simulink model "unrolled_pipelined_parallel"  (R2015b)
settings: Solver=FixedStepDiscrete  SolverMode=SingleTasking  StartTime=0.0  StopTime=10.0  RelTol=1e-3
undefined symbols (not defined in the file or in its folder): a, b
libraries: shlslibv1 x8781
(part 14 of 32)

== system unrolled_pipelined_parallel/Subsystem/Subsystem3/SB_rs_MIX_COLUMN/Subsystem2/multby2 ==
  In1 : Inport
  Binary Logic : shlslibv1/Math Functions/Binary Logic  syn_binlog_exp=a^b  synBlockType=primitive  synLatency=0  synBlockId=13
  Comparator : shlslibv1/Math Functions/Comparator  syn_comp_opr=a==b  syn_comp_const=off  syn_comp_val=0  syn_en_se=off  synBlockType=primitive  synLatency=0  synBlockId=14
  Constant : shlslibv1/Sources/Constant  syn_cst_val=1  syn_cst_format=Automatic  syn_cst_wl=1  syn_cst_fl=0  syn_cst_dt=unsigned  syn_cst_rnd=on  syn_cst_st=-1  synBlockType=primitive  synLatency=0  synBlockId=15
  Constant1 : shlslibv1/Sources/Constant  syn_cst_val=1  syn_cst_format=Automatic  syn_cst_wl=1  syn_cst_fl=0  syn_cst_dt=unsigned  syn_cst_rnd=on  syn_cst_st=-1  synBlockType=primitive  synLatency=0  synBlockId=15
  Constant2 : shlslibv1/Sources/Constant  syn_cst_val=27  syn_cst_format=Specify  syn_cst_wl=8  syn_cst_fl=0  syn_cst_dt=unsigned  syn_cst_rnd=on  syn_cst_st=-1  synBlockType=primitive  synLatency=0  synBlockId=15
  Extract : shlslibv1/Signal Operations/Extract  syn_extract_vec=[7]  synBlockType=primitive  synLatency=0  synBlockId=17
  Mux : shlslibv1/Signal Operations/Mux  syn_in_nb=2  syn_out_f=Full Precision  syn_out_wl=16  syn_out_fl=8  syn_out_dt=signed  syn_en_se=off  synBlockType=primitive  synLatency=0  synBlockId=16
  Shifter : shlslibv1/Math Functions/Shifter  syn_shifter_opr=<<  syn_out_f=Automatic  syn_out_wl=16  syn_out_fl=8  syn_out_dt=signed  synBlockType=primitive  synLatency=0  synBlockId=12
  Out1 : Outport
  wires:
  Extract/1 -> Comparator/1
  In1/1 -> Shifter/1, Extract/1
  Constant/1 -> Shifter/2
  Constant1/1 -> Comparator/2
  Shifter/1 -> Mux/2, Binary Logic/1
  Comparator/1 -> Mux/1
  Mux/1 -> Out1/1
  Binary Logic/1 -> Mux/3
  Constant2/1 -> Binary Logic/2

== system unrolled_pipelined_parallel/Subsystem/Subsystem3/SB_rs_MIX_COLUMN/Subsystem2/multby3 ==
  In1 : Inport
  Binary Logic : shlslibv1/Math Functions/Binary Logic  syn_binlog_exp=a^b  synBlockType=primitive  synLatency=0  synBlockId=13
  Comparator : shlslibv1/Math Functions/Comparator  syn_comp_opr=a==b  syn_comp_const=off  syn_comp_val=0  syn_en_se=off  synBlockType=primitive  synLatency=0  synBlockId=14
  Constant : shlslibv1/Sources/Constant  syn_cst_val=1  syn_cst_format=Automatic  syn_cst_wl=1  syn_cst_fl=0  syn_cst_dt=unsigned  syn_cst_rnd=on  syn_cst_st=-1  synBlockType=primitive  synLatency=0  synBlockId=15
  Constant1 : shlslibv1/Sources/Constant  syn_cst_val=1  syn_cst_format=Automatic  syn_cst_wl=1  syn_cst_fl=0  syn_cst_dt=unsigned  syn_cst_rnd=on  syn_cst_st=-1  synBlockType=primitive  synLatency=0  synBlockId=15
  Constant2 : shlslibv1/Sources/Constant  syn_cst_val=27  syn_cst_format=Specify  syn_cst_wl=8  syn_cst_fl=0  syn_cst_dt=unsigned  syn_cst_rnd=on  syn_cst_st=-1  synBlockType=primitive  synLatency=0  synBlockId=15
  Extract : shlslibv1/Signal Operations/Extract  syn_extract_vec=[7]  synBlockType=primitive  synLatency=0  synBlockId=17
  Mux : shlslibv1/Signal Operations/Mux  syn_in_nb=2  syn_out_f=Full Precision  syn_out_wl=16  syn_out_fl=8  syn_out_dt=signed  syn_en_se=off  synBlockType=primitive  synLatency=0  synBlockId=16
  Shifter : shlslibv1/Math Functions/Shifter  syn_shifter_opr=<<  syn_out_f=Automatic  syn_out_wl=16  syn_out_fl=8  syn_out_dt=signed  synBlockType=primitive  synLatency=0  synBlockId=12
  Out1 : Outport
  wires:
  Extract/1 -> Comparator/1
  In1/1 -> Shifter/1, Extract/1
  Constant/1 -> Shifter/2
  Constant1/1 -> Comparator/2
  Shifter/1 -> Mux/2, Binary Logic/1
  Comparator/1 -> Mux/1
  Mux/1 -> Out1/1
  Binary Logic/1 -> Mux/3
  Constant2/1 -> Binary Logic/2

== system unrolled_pipelined_parallel/Subsystem/Subsystem3/SB_rs_MIX_COLUMN/Subsystem2/multby4 ==
  In1 : Inport
  Binary Logic : shlslibv1/Math Functions/Binary Logic  syn_binlog_exp=a^b  synBlockType=primitive  synLatency=0  synBlockId=13
  Comparator : shlslibv1/Math Functions/Comparator  syn_comp_opr=a==b  syn_comp_const=off  syn_comp_val=0  syn_en_se=off  synBlockType=primitive  synLatency=0  synBlockId=14
  Constant : shlslibv1/Sources/Constant  syn_cst_val=1  syn_cst_format=Automatic  syn_cst_wl=1  syn_cst_fl=0  syn_cst_dt=unsigned  syn_cst_rnd=on  syn_cst_st=-1  synBlockType=primitive  synLatency=0  synBlockId=15
  Constant1 : shlslibv1/Sources/Constant  syn_cst_val=1  syn_cst_format=Automatic  syn_cst_wl=1  syn_cst_fl=0  syn_cst_dt=unsigned  syn_cst_rnd=on  syn_cst_st=-1  synBlockType=primitive  synLatency=0  synBlockId=15
  Constant2 : shlslibv1/Sources/Constant  syn_cst_val=27  syn_cst_format=Specify  syn_cst_wl=8  syn_cst_fl=0  syn_cst_dt=unsigned  syn_cst_rnd=on  syn_cst_st=-1  synBlockType=primitive  synLatency=0  synBlockId=15
  Extract : shlslibv1/Signal Operations/Extract  syn_extract_vec=[7]  synBlockType=primitive  synLatency=0  synBlockId=17
  Mux : shlslibv1/Signal Operations/Mux  syn_in_nb=2  syn_out_f=Full Precision  syn_out_wl=16  syn_out_fl=8  syn_out_dt=signed  syn_en_se=off  synBlockType=primitive  synLatency=0  synBlockId=16
  Shifter : shlslibv1/Math Functions/Shifter  syn_shifter_opr=<<  syn_out_f=Automatic  syn_out_wl=16  syn_out_fl=8  syn_out_dt=signed  synBlockType=primitive  synLatency=0  synBlockId=12
  Out1 : Outport
  wires:
  Extract/1 -> Comparator/1
  In1/1 -> Shifter/1, Extract/1
  Constant/1 -> Shifter/2
  Constant1/1 -> Comparator/2
  Shifter/1 -> Mux/2, Binary Logic/1
  Comparator/1 -> Mux/1
  Mux/1 -> Out1/1
  Binary Logic/1 -> Mux/3
  Constant2/1 -> Binary Logic/2

== system unrolled_pipelined_parallel/Subsystem/Subsystem3/SB_rs_MIX_COLUMN/Subsystem2/multby5 ==
  In1 : Inport
  Binary Logic : shlslibv1/Math Functions/Binary Logic  syn_binlog_exp=a^b  synBlockType=primitive  synLatency=0  synBlockId=13
  Comparator : shlslibv1/Math Functions/Comparator  syn_comp_opr=a==b  syn_comp_const=off  syn_comp_val=0  syn_en_se=off  synBlockType=primitive  synLatency=0  synBlockId=14
  Constant : shlslibv1/Sources/Constant  syn_cst_val=1  syn_cst_format=Automatic  syn_cst_wl=1  syn_cst_fl=0  syn_cst_dt=unsigned  syn_cst_rnd=on  syn_cst_st=-1  synBlockType=primitive  synLatency=0  synBlockId=15
  Constant1 : shlslibv1/Sources/Constant  syn_cst_val=1  syn_cst_format=Automatic  syn_cst_wl=1  syn_cst_fl=0  syn_cst_dt=unsigned  syn_cst_rnd=on  syn_cst_st=-1  synBlockType=primitive  synLatency=0  synBlockId=15
  Constant2 : shlslibv1/Sources/Constant  syn_cst_val=27  syn_cst_format=Specify  syn_cst_wl=8  syn_cst_fl=0  syn_cst_dt=unsigned  syn_cst_rnd=on  syn_cst_st=-1  synBlockType=primitive  synLatency=0  synBlockId=15
  Extract : shlslibv1/Signal Operations/Extract  syn_extract_vec=[7]  synBlockType=primitive  synLatency=0  synBlockId=17
  Mux : shlslibv1/Signal Operations/Mux  syn_in_nb=2  syn_out_f=Full Precision  syn_out_wl=16  syn_out_fl=8  syn_out_dt=signed  syn_en_se=off  synBlockType=primitive  synLatency=0  synBlockId=16
  Shifter : shlslibv1/Math Functions/Shifter  syn_shifter_opr=<<  syn_out_f=Automatic  syn_out_wl=16  syn_out_fl=8  syn_out_dt=signed  synBlockType=primitive  synLatency=0  synBlockId=12
  Out1 : Outport
  wires:
  Extract/1 -> Comparator/1
  In1/1 -> Shifter/1, Extract/1
  Constant/1 -> Shifter/2
  Constant1/1 -> Comparator/2
  Shifter/1 -> Mux/2, Binary Logic/1
  Comparator/1 -> Mux/1
  Mux/1 -> Out1/1
  Binary Logic/1 -> Mux/3
  Constant2/1 -> Binary Logic/2

== system unrolled_pipelined_parallel/Subsystem/Subsystem3/SB_rs_MIX_COLUMN/Subsystem2/multby6 ==
  In1 : Inport
  Binary Logic : shlslibv1/Math Functions/Binary Logic  syn_binlog_exp=a^b  synBlockType=primitive  synLatency=0  synBlockId=13
  Comparator : shlslibv1/Math Functions/Comparator  syn_comp_opr=a==b  syn_comp_const=off  syn_comp_val=0  syn_en_se=off  synBlockType=primitive  synLatency=0  synBlockId=14
  Constant : shlslibv1/Sources/Constant  syn_cst_val=1  syn_cst_format=Automatic  syn_cst_wl=1  syn_cst_fl=0  syn_cst_dt=unsigned  syn_cst_rnd=on  syn_cst_st=-1  synBlockType=primitive  synLatency=0  synBlockId=15
  Constant1 : shlslibv1/Sources/Constant  syn_cst_val=1  syn_cst_format=Automatic  syn_cst_wl=1  syn_cst_fl=0  syn_cst_dt=unsigned  syn_cst_rnd=on  syn_cst_st=-1  synBlockType=primitive  synLatency=0  synBlockId=15
  Constant2 : shlslibv1/Sources/Constant  syn_cst_val=27  syn_cst_format=Specify  syn_cst_wl=8  syn_cst_fl=0  syn_cst_dt=unsigned  syn_cst_rnd=on  syn_cst_st=-1  synBlockType=primitive  synLatency=0  synBlockId=15
  Extract : shlslibv1/Signal Operations/Extract  syn_extract_vec=[7]  synBlockType=primitive  synLatency=0  synBlockId=17
  Mux : shlslibv1/Signal Operations/Mux  syn_in_nb=2  syn_out_f=Full Precision  syn_out_wl=16  syn_out_fl=8  syn_out_dt=signed  syn_en_se=off  synBlockType=primitive  synLatency=0  synBlockId=16
  Shifter : shlslibv1/Math Functions/Shifter  syn_shifter_opr=<<  syn_out_f=Automatic  syn_out_wl=16  syn_out_fl=8  syn_out_dt=signed  synBlockType=primitive  synLatency=0  synBlockId=12
  Out1 : Outport
  wires:
  Extract/1 -> Comparator/1
  In1/1 -> Shifter/1, Extract/1
  Constant/1 -> Shifter/2
  Constant1/1 -> Comparator/2
  Shifter/1 -> Mux/2, Binary Logic/1
  Comparator/1 -> Mux/1
  Mux/1 -> Out1/1
  Binary Logic/1 -> Mux/3
  Constant2/1 -> Binary Logic/2

== system unrolled_pipelined_parallel/Subsystem/Subsystem3/SB_rs_MIX_COLUMN/Subsystem2/multby7 ==
  In1 : Inport
  Binary Logic : shlslibv1/Math Functions/Binary Logic  syn_binlog_exp=a^b  synBlockType=primitive  synLatency=0  synBlockId=13
  Comparator : shlslibv1/Math Functions/Comparator  syn_comp_opr=a==b  syn_comp_const=off  syn_comp_val=0  syn_en_se=off  synBlockType=primitive  synLatency=0  synBlockId=14
  Constant : shlslibv1/Sources/Constant  syn_cst_val=1  syn_cst_format=Automatic  syn_cst_wl=1  syn_cst_fl=0  syn_cst_dt=unsigned  syn_cst_rnd=on  syn_cst_st=-1  synBlockType=primitive  synLatency=0  synBlockId=15
  Constant1 : shlslibv1/Sources/Constant  syn_cst_val=1  syn_cst_format=Automatic  syn_cst_wl=1  syn_cst_fl=0  syn_cst_dt=unsigned  syn_cst_rnd=on  syn_cst_st=-1  synBlockType=primitive  synLatency=0  synBlockId=15
  Constant2 : shlslibv1/Sources/Constant  syn_cst_val=27  syn_cst_format=Specify  syn_cst_wl=8  syn_cst_fl=0  syn_cst_dt=unsigned  syn_cst_rnd=on  syn_cst_st=-1  synBlockType=primitive  synLatency=0  synBlockId=15
  Extract : shlslibv1/Signal Operations/Extract  syn_extract_vec=[7]  synBlockType=primitive  synLatency=0  synBlockId=17
  Mux : shlslibv1/Signal Operations/Mux  syn_in_nb=2  syn_out_f=Full Precision  syn_out_wl=16  syn_out_fl=8  syn_out_dt=signed  syn_en_se=off  synBlockType=primitive  synLatency=0  synBlockId=16
  Shifter : shlslibv1/Math Functions/Shifter  syn_shifter_opr=<<  syn_out_f=Automatic  syn_out_wl=16  syn_out_fl=8  syn_out_dt=signed  synBlockType=primitive  synLatency=0  synBlockId=12
  Out1 : Outport
  wires:
  Extract/1 -> Comparator/1
  In1/1 -> Shifter/1, Extract/1
  Constant/1 -> Shifter/2
  Constant1/1 -> Comparator/2
  Shifter/1 -> Mux/2, Binary Logic/1
  Comparator/1 -> Mux/1
  Mux/1 -> Out1/1
  Binary Logic/1 -> Mux/3
  Constant2/1 -> Binary Logic/2

== system unrolled_pipelined_parallel/Subsystem/Subsystem3/SB_rs_MIX_COLUMN/Subsystem2/multby8 ==
  In1 : Inport
  Binary Logic : shlslibv1/Math Functions/Binary Logic  syn_binlog_exp=a^b  synBlockType=primitive  synLatency=0  synBlockId=13
  Comparator : shlslibv1/Math Functions/Comparator  syn_comp_opr=a==b  syn_comp_const=off  syn_comp_val=0  syn_en_se=off  synBlockType=primitive  synLatency=0  synBlockId=14
  Constant : shlslibv1/Sources/Constant  syn_cst_val=1  syn_cst_format=Automatic  syn_cst_wl=1  syn_cst_fl=0  syn_cst_dt=unsigned  syn_cst_rnd=on  syn_cst_st=-1  synBlockType=primitive  synLatency=0  synBlockId=15
  Constant1 : shlslibv1/Sources/Constant  syn_cst_val=1  syn_cst_format=Automatic  syn_cst_wl=1  syn_cst_fl=0  syn_cst_dt=unsigned  syn_cst_rnd=on  syn_cst_st=-1  synBlockType=primitive  synLatency=0  synBlockId=15
  Constant2 : shlslibv1/Sources/Constant  syn_cst_val=27  syn_cst_format=Specify  syn_cst_wl=8  syn_cst_fl=0  syn_cst_dt=unsigned  syn_cst_rnd=on  syn_cst_st=-1  synBlockType=primitive  synLatency=0  synBlockId=15
  Extract : shlslibv1/Signal Operations/Extract  syn_extract_vec=[7]  synBlockType=primitive  synLatency=0  synBlockId=17
  Mux : shlslibv1/Signal Operations/Mux  syn_in_nb=2  syn_out_f=Full Precision  syn_out_wl=16  syn_out_fl=8  syn_out_dt=signed  syn_en_se=off  synBlockType=primitive  synLatency=0  synBlockId=16
  Shifter : shlslibv1/Math Functions/Shifter  syn_shifter_opr=<<  syn_out_f=Automatic  syn_out_wl=16  syn_out_fl=8  syn_out_dt=signed  synBlockType=primitive  synLatency=0  synBlockId=12
  Out1 : Outport
  wires:
  Extract/1 -> Comparator/1
  In1/1 -> Shifter/1, Extract/1
  Constant/1 -> Shifter/2
  Constant1/1 -> Comparator/2
  Shifter/1 -> Mux/2, Binary Logic/1
  Comparator/1 -> Mux/1
  Mux/1 -> Out1/1
  Binary Logic/1 -> Mux/3
  Constant2/1 -> Binary Logic/2

== system unrolled_pipelined_parallel/Subsystem/Subsystem3/SB_rs_MIX_COLUMN/Subsystem3/multby1 ==
  In1 : Inport
  Binary Logic : shlslibv1/Math Functions/Binary Logic  syn_binlog_exp=a^b  synBlockType=primitive  synLatency=0  synBlockId=13
  Comparator : shlslibv1/Math Functions/Comparator  syn_comp_opr=a==b  syn_comp_const=off  syn_comp_val=0  syn_en_se=off  synBlockType=primitive  synLatency=0  synBlockId=14
  Constant : shlslibv1/Sources/Constant  syn_cst_val=1  syn_cst_format=Automatic  syn_cst_wl=1  syn_cst_fl=0  syn_cst_dt=unsigned  syn_cst_rnd=on  syn_cst_st=-1  synBlockType=primitive  synLatency=0  synBlockId=15
  Constant1 : shlslibv1/Sources/Constant  syn_cst_val=1  syn_cst_format=Automatic  syn_cst_wl=1  syn_cst_fl=0  syn_cst_dt=unsigned  syn_cst_rnd=on  syn_cst_st=-1  synBlockType=primitive  synLatency=0  synBlockId=15
  Constant2 : shlslibv1/Sources/Constant  syn_cst_val=27  syn_cst_format=Specify  syn_cst_wl=8  syn_cst_fl=0  syn_cst_dt=unsigned  syn_cst_rnd=on  syn_cst_st=-1  synBlockType=primitive  synLatency=0  synBlockId=15
  Extract : shlslibv1/Signal Operations/Extract  syn_extract_vec=[7]  synBlockType=primitive  synLatency=0  synBlockId=17
  Mux : shlslibv1/Signal Operations/Mux  syn_in_nb=2  syn_out_f=Full Precision  syn_out_wl=16  syn_out_fl=8  syn_out_dt=signed  syn_en_se=off  synBlockType=primitive  synLatency=0  synBlockId=16
  Shifter : shlslibv1/Math Functions/Shifter  syn_shifter_opr=<<  syn_out_f=Automatic  syn_out_wl=16  syn_out_fl=8  syn_out_dt=signed  synBlockType=primitive  synLatency=0  synBlockId=12
  Out1 : Outport
  wires:
  Extract/1 -> Comparator/1
  In1/1 -> Shifter/1, Extract/1
  Constant/1 -> Shifter/2
  Constant1/1 -> Comparator/2
  Shifter/1 -> Mux/2, Binary Logic/1
  Comparator/1 -> Mux/1
  Mux/1 -> Out1/1
  Binary Logic/1 -> Mux/3
  Constant2/1 -> Binary Logic/2

== system unrolled_pipelined_parallel/Subsystem/Subsystem3/SB_rs_MIX_COLUMN/Subsystem3/multby2 ==
  In1 : Inport
  Binary Logic : shlslibv1/Math Functions/Binary Logic  syn_binlog_exp=a^b  synBlockType=primitive  synLatency=0  synBlockId=13
  Comparator : shlslibv1/Math Functions/Comparator  syn_comp_opr=a==b  syn_comp_const=off  syn_comp_val=0  syn_en_se=off  synBlockType=primitive  synLatency=0  synBlockId=14
  Constant : shlslibv1/Sources/Constant  syn_cst_val=1  syn_cst_format=Automatic  syn_cst_wl=1  syn_cst_fl=0  syn_cst_dt=unsigned  syn_cst_rnd=on  syn_cst_st=-1  synBlockType=primitive  synLatency=0  synBlockId=15
  Constant1 : shlslibv1/Sources/Constant  syn_cst_val=1  syn_cst_format=Automatic  syn_cst_wl=1  syn_cst_fl=0  syn_cst_dt=unsigned  syn_cst_rnd=on  syn_cst_st=-1  synBlockType=primitive  synLatency=0  synBlockId=15
  Constant2 : shlslibv1/Sources/Constant  syn_cst_val=27  syn_cst_format=Specify  syn_cst_wl=8  syn_cst_fl=0  syn_cst_dt=unsigned  syn_cst_rnd=on  syn_cst_st=-1  synBlockType=primitive  synLatency=0  synBlockId=15
  Extract : shlslibv1/Signal Operations/Extract  syn_extract_vec=[7]  synBlockType=primitive  synLatency=0  synBlockId=17
  Mux : shlslibv1/Signal Operations/Mux  syn_in_nb=2  syn_out_f=Full Precision  syn_out_wl=16  syn_out_fl=8  syn_out_dt=signed  syn_en_se=off  synBlockType=primitive  synLatency=0  synBlockId=16
  Shifter : shlslibv1/Math Functions/Shifter  syn_shifter_opr=<<  syn_out_f=Automatic  syn_out_wl=16  syn_out_fl=8  syn_out_dt=signed  synBlockType=primitive  synLatency=0  synBlockId=12
  Out1 : Outport
  wires:
  Extract/1 -> Comparator/1
  In1/1 -> Shifter/1, Extract/1
  Constant/1 -> Shifter/2
  Constant1/1 -> Comparator/2
  Shifter/1 -> Mux/2, Binary Logic/1
  Comparator/1 -> Mux/1
  Mux/1 -> Out1/1
  Binary Logic/1 -> Mux/3
  Constant2/1 -> Binary Logic/2

== system unrolled_pipelined_parallel/Subsystem/Subsystem3/SB_rs_MIX_COLUMN/Subsystem3/multby3 ==
  In1 : Inport
  Binary Logic : shlslibv1/Math Functions/Binary Logic  syn_binlog_exp=a^b  synBlockType=primitive  synLatency=0  synBlockId=13
  Comparator : shlslibv1/Math Functions/Comparator  syn_comp_opr=a==b  syn_comp_const=off  syn_comp_val=0  syn_en_se=off  synBlockType=primitive  synLatency=0  synBlockId=14
  Constant : shlslibv1/Sources/Constant  syn_cst_val=1  syn_cst_format=Automatic  syn_cst_wl=1  syn_cst_fl=0  syn_cst_dt=unsigned  syn_cst_rnd=on  syn_cst_st=-1  synBlockType=primitive  synLatency=0  synBlockId=15
  Constant1 : shlslibv1/Sources/Constant  syn_cst_val=1  syn_cst_format=Automatic  syn_cst_wl=1  syn_cst_fl=0  syn_cst_dt=unsigned  syn_cst_rnd=on  syn_cst_st=-1  synBlockType=primitive  synLatency=0  synBlockId=15
  Constant2 : shlslibv1/Sources/Constant  syn_cst_val=27  syn_cst_format=Specify  syn_cst_wl=8  syn_cst_fl=0  syn_cst_dt=unsigned  syn_cst_rnd=on  syn_cst_st=-1  synBlockType=primitive  synLatency=0  synBlockId=15
  Extract : shlslibv1/Signal Operations/Extract  syn_extract_vec=[7]  synBlockType=primitive  synLatency=0  synBlockId=17
  Mux : shlslibv1/Signal Operations/Mux  syn_in_nb=2  syn_out_f=Full Precision  syn_out_wl=16  syn_out_fl=8  syn_out_dt=signed  syn_en_se=off  synBlockType=primitive  synLatency=0  synBlockId=16
  Shifter : shlslibv1/Math Functions/Shifter  syn_shifter_opr=<<  syn_out_f=Automatic  syn_out_wl=16  syn_out_fl=8  syn_out_dt=signed  synBlockType=primitive  synLatency=0  synBlockId=12
  Out1 : Outport
  wires:
  Extract/1 -> Comparator/1
  In1/1 -> Shifter/1, Extract/1
  Constant/1 -> Shifter/2
  Constant1/1 -> Comparator/2
  Shifter/1 -> Mux/2, Binary Logic/1
  Comparator/1 -> Mux/1
  Mux/1 -> Out1/1
  Binary Logic/1 -> Mux/3
  Constant2/1 -> Binary Logic/2

== system unrolled_pipelined_parallel/Subsystem/Subsystem3/SB_rs_MIX_COLUMN/Subsystem3/multby4 ==
  In1 : Inport
  Binary Logic : shlslibv1/Math Functions/Binary Logic  syn_binlog_exp=a^b  synBlockType=primitive  synLatency=0  synBlockId=13
  Comparator : shlslibv1/Math Functions/Comparator  syn_comp_opr=a==b  syn_comp_const=off  syn_comp_val=0  syn_en_se=off  synBlockType=primitive  synLatency=0  synBlockId=14
  Constant : shlslibv1/Sources/Constant  syn_cst_val=1  syn_cst_format=Automatic  syn_cst_wl=1  syn_cst_fl=0  syn_cst_dt=unsigned  syn_cst_rnd=on  syn_cst_st=-1  synBlockType=primitive  synLatency=0  synBlockId=15
  Constant1 : shlslibv1/Sources/Constant  syn_cst_val=1  syn_cst_format=Automatic  syn_cst_wl=1  syn_cst_fl=0  syn_cst_dt=unsigned  syn_cst_rnd=on  syn_cst_st=-1  synBlockType=primitive  synLatency=0  synBlockId=15
  Constant2 : shlslibv1/Sources/Constant  syn_cst_val=27  syn_cst_format=Specify  syn_cst_wl=8  syn_cst_fl=0  syn_cst_dt=unsigned  syn_cst_rnd=on  syn_cst_st=-1  synBlockType=primitive  synLatency=0  synBlockId=15
  Extract : shlslibv1/Signal Operations/Extract  syn_extract_vec=[7]  synBlockType=primitive  synLatency=0  synBlockId=17
  Mux : shlslibv1/Signal Operations/Mux  syn_in_nb=2  syn_out_f=Full Precision  syn_out_wl=16  syn_out_fl=8  syn_out_dt=signed  syn_en_se=off  synBlockType=primitive  synLatency=0  synBlockId=16
  Shifter : shlslibv1/Math Functions/Shifter  syn_shifter_opr=<<  syn_out_f=Automatic  syn_out_wl=16  syn_out_fl=8  syn_out_dt=signed  synBlockType=primitive  synLatency=0  synBlockId=12
  Out1 : Outport
  wires:
  Extract/1 -> Comparator/1
  In1/1 -> Shifter/1, Extract/1
  Constant/1 -> Shifter/2
  Constant1/1 -> Comparator/2
  Shifter/1 -> Mux/2, Binary Logic/1
  Comparator/1 -> Mux/1
  Mux/1 -> Out1/1
  Binary Logic/1 -> Mux/3
  Constant2/1 -> Binary Logic/2

== system unrolled_pipelined_parallel/Subsystem/Subsystem3/SB_rs_MIX_COLUMN/Subsystem3/multby5 ==
  In1 : Inport
  Binary Logic : shlslibv1/Math Functions/Binary Logic  syn_binlog_exp=a^b  synBlockType=primitive  synLatency=0  synBlockId=13
  Comparator : shlslibv1/Math Functions/Comparator  syn_comp_opr=a==b  syn_comp_const=off  syn_comp_val=0  syn_en_se=off  synBlockType=primitive  synLatency=0  synBlockId=14
  Constant : shlslibv1/Sources/Constant  syn_cst_val=1  syn_cst_format=Automatic  syn_cst_wl=1  syn_cst_fl=0  syn_cst_dt=unsigned  syn_cst_rnd=on  syn_cst_st=-1  synBlockType=primitive  synLatency=0  synBlockId=15
  Constant1 : shlslibv1/Sources/Constant  syn_cst_val=1  syn_cst_format=Automatic  syn_cst_wl=1  syn_cst_fl=0  syn_cst_dt=unsigned  syn_cst_rnd=on  syn_cst_st=-1  synBlockType=primitive  synLatency=0  synBlockId=15
  Constant2 : shlslibv1/Sources/Constant  syn_cst_val=27  syn_cst_format=Specify  syn_cst_wl=8  syn_cst_fl=0  syn_cst_dt=unsigned  syn_cst_rnd=on  syn_cst_st=-1  synBlockType=primitive  synLatency=0  synBlockId=15
  Extract : shlslibv1/Signal Operations/Extract  syn_extract_vec=[7]  synBlockType=primitive  synLatency=0  synBlockId=17
  Mux : shlslibv1/Signal Operations/Mux  syn_in_nb=2  syn_out_f=Full Precision  syn_out_wl=16  syn_out_fl=8  syn_out_dt=signed  syn_en_se=off  synBlockType=primitive  synLatency=0  synBlockId=16
  Shifter : shlslibv1/Math Functions/Shifter  syn_shifter_opr=<<  syn_out_f=Automatic  syn_out_wl=16  syn_out_fl=8  syn_out_dt=signed  synBlockType=primitive  synLatency=0  synBlockId=12
  Out1 : Outport
  wires:
  Extract/1 -> Comparator/1
  In1/1 -> Shifter/1, Extract/1
  Constant/1 -> Shifter/2
  Constant1/1 -> Comparator/2
  Shifter/1 -> Mux/2, Binary Logic/1
  Comparator/1 -> Mux/1
  Mux/1 -> Out1/1
  Binary Logic/1 -> Mux/3
  Constant2/1 -> Binary Logic/2

== system unrolled_pipelined_parallel/Subsystem/Subsystem3/SB_rs_MIX_COLUMN/Subsystem3/multby6 ==
  In1 : Inport
  Binary Logic : shlslibv1/Math Functions/Binary Logic  syn_binlog_exp=a^b  synBlockType=primitive  synLatency=0  synBlockId=13
  Comparator : shlslibv1/Math Functions/Comparator  syn_comp_opr=a==b  syn_comp_const=off  syn_comp_val=0  syn_en_se=off  synBlockType=primitive  synLatency=0  synBlockId=14
  Constant : shlslibv1/Sources/Constant  syn_cst_val=1  syn_cst_format=Automatic  syn_cst_wl=1  syn_cst_fl=0  syn_cst_dt=unsigned  syn_cst_rnd=on  syn_cst_st=-1  synBlockType=primitive  synLatency=0  synBlockId=15
  Constant1 : shlslibv1/Sources/Constant  syn_cst_val=1  syn_cst_format=Automatic  syn_cst_wl=1  syn_cst_fl=0  syn_cst_dt=unsigned  syn_cst_rnd=on  syn_cst_st=-1  synBlockType=primitive  synLatency=0  synBlockId=15
  Constant2 : shlslibv1/Sources/Constant  syn_cst_val=27  syn_cst_format=Specify  syn_cst_wl=8  syn_cst_fl=0  syn_cst_dt=unsigned  syn_cst_rnd=on  syn_cst_st=-1  synBlockType=primitive  synLatency=0  synBlockId=15
  Extract : shlslibv1/Signal Operations/Extract  syn_extract_vec=[7]  synBlockType=primitive  synLatency=0  synBlockId=17
  Mux : shlslibv1/Signal Operations/Mux  syn_in_nb=2  syn_out_f=Full Precision  syn_out_wl=16  syn_out_fl=8  syn_out_dt=signed  syn_en_se=off  synBlockType=primitive  synLatency=0  synBlockId=16
  Shifter : shlslibv1/Math Functions/Shifter  syn_shifter_opr=<<  syn_out_f=Automatic  syn_out_wl=16  syn_out_fl=8  syn_out_dt=signed  synBlockType=primitive  synLatency=0  synBlockId=12
  Out1 : Outport
  wires:
  Extract/1 -> Comparator/1
  In1/1 -> Shifter/1, Extract/1
  Constant/1 -> Shifter/2
  Constant1/1 -> Comparator/2
  Shifter/1 -> Mux/2, Binary Logic/1
  Comparator/1 -> Mux/1
  Mux/1 -> Out1/1
  Binary Logic/1 -> Mux/3
  Constant2/1 -> Binary Logic/2

== system unrolled_pipelined_parallel/Subsystem/Subsystem3/SB_rs_MIX_COLUMN/Subsystem3/multby7 ==
  In1 : Inport
  Binary Logic : shlslibv1/Math Functions/Binary Logic  syn_binlog_exp=a^b  synBlockType=primitive  synLatency=0  synBlockId=13
  Comparator : shlslibv1/Math Functions/Comparator  syn_comp_opr=a==b  syn_comp_const=off  syn_comp_val=0  syn_en_se=off  synBlockType=primitive  synLatency=0  synBlockId=14
  Constant : shlslibv1/Sources/Constant  syn_cst_val=1  syn_cst_format=Automatic  syn_cst_wl=1  syn_cst_fl=0  syn_cst_dt=unsigned  syn_cst_rnd=on  syn_cst_st=-1  synBlockType=primitive  synLatency=0  synBlockId=15
  Constant1 : shlslibv1/Sources/Constant  syn_cst_val=1  syn_cst_format=Automatic  syn_cst_wl=1  syn_cst_fl=0  syn_cst_dt=unsigned  syn_cst_rnd=on  syn_cst_st=-1  synBlockType=primitive  synLatency=0  synBlockId=15
  Constant2 : shlslibv1/Sources/Constant  syn_cst_val=27  syn_cst_format=Specify  syn_cst_wl=8  syn_cst_fl=0  syn_cst_dt=unsigned  syn_cst_rnd=on  syn_cst_st=-1  synBlockType=primitive  synLatency=0  synBlockId=15
  Extract : shlslibv1/Signal Operations/Extract  syn_extract_vec=[7]  synBlockType=primitive  synLatency=0  synBlockId=17
  Mux : shlslibv1/Signal Operations/Mux  syn_in_nb=2  syn_out_f=Full Precision  syn_out_wl=16  syn_out_fl=8  syn_out_dt=signed  syn_en_se=off  synBlockType=primitive  synLatency=0  synBlockId=16
  Shifter : shlslibv1/Math Functions/Shifter  syn_shifter_opr=<<  syn_out_f=Automatic  syn_out_wl=16  syn_out_fl=8  syn_out_dt=signed  synBlockType=primitive  synLatency=0  synBlockId=12
  Out1 : Outport
  wires:
  Extract/1 -> Comparator/1
  In1/1 -> Shifter/1, Extract/1
  Constant/1 -> Shifter/2
  Constant1/1 -> Comparator/2
  Shifter/1 -> Mux/2, Binary Logic/1
  Comparator/1 -> Mux/1
  Mux/1 -> Out1/1
  Binary Logic/1 -> Mux/3
  Constant2/1 -> Binary Logic/2

== system unrolled_pipelined_parallel/Subsystem/Subsystem3/SB_rs_MIX_COLUMN/Subsystem3/multby8 ==
  In1 : Inport
  Binary Logic : shlslibv1/Math Functions/Binary Logic  syn_binlog_exp=a^b  synBlockType=primitive  synLatency=0  synBlockId=13
  Comparator : shlslibv1/Math Functions/Comparator  syn_comp_opr=a==b  syn_comp_const=off  syn_comp_val=0  syn_en_se=off  synBlockType=primitive  synLatency=0  synBlockId=14
  Constant : shlslibv1/Sources/Constant  syn_cst_val=1  syn_cst_format=Automatic  syn_cst_wl=1  syn_cst_fl=0  syn_cst_dt=unsigned  syn_cst_rnd=on  syn_cst_st=-1  synBlockType=primitive  synLatency=0  synBlockId=15
  Constant1 : shlslibv1/Sources/Constant  syn_cst_val=1  syn_cst_format=Automatic  syn_cst_wl=1  syn_cst_fl=0  syn_cst_dt=unsigned  syn_cst_rnd=on  syn_cst_st=-1  synBlockType=primitive  synLatency=0  synBlockId=15
  Constant2 : shlslibv1/Sources/Constant  syn_cst_val=27  syn_cst_format=Specify  syn_cst_wl=8  syn_cst_fl=0  syn_cst_dt=unsigned  syn_cst_rnd=on  syn_cst_st=-1  synBlockType=primitive  synLatency=0  synBlockId=15
  Extract : shlslibv1/Signal Operations/Extract  syn_extract_vec=[7]  synBlockType=primitive  synLatency=0  synBlockId=17
  Mux : shlslibv1/Signal Operations/Mux  syn_in_nb=2  syn_out_f=Full Precision  syn_out_wl=16  syn_out_fl=8  syn_out_dt=signed  syn_en_se=off  synBlockType=primitive  synLatency=0  synBlockId=16
  Shifter : shlslibv1/Math Functions/Shifter  syn_shifter_opr=<<  syn_out_f=Automatic  syn_out_wl=16  syn_out_fl=8  syn_out_dt=signed  synBlockType=primitive  synLatency=0  synBlockId=12
  Out1 : Outport
  wires:
  Extract/1 -> Comparator/1
  In1/1 -> Shifter/1, Extract/1
  Constant/1 -> Shifter/2
  Constant1/1 -> Comparator/2
  Shifter/1 -> Mux/2, Binary Logic/1
  Comparator/1 -> Mux/1
  Mux/1 -> Out1/1
  Binary Logic/1 -> Mux/3
  Constant2/1 -> Binary Logic/2

== system unrolled_pipelined_parallel/Subsystem/Subsystem4/SB_rs_MIX_COLUMN/Subsystem/multby1 ==
  In1 : Inport
  Binary Logic : shlslibv1/Math Functions/Binary Logic  syn_binlog_exp=a^b  synBlockType=primitive  synLatency=0  synBlockId=13
  Comparator : shlslibv1/Math Functions/Comparator  syn_comp_opr=a==b  syn_comp_const=off  syn_comp_val=0  syn_en_se=off  synBlockType=primitive  synLatency=0  synBlockId=14
  Constant : shlslibv1/Sources/Constant  syn_cst_val=1  syn_cst_format=Automatic  syn_cst_wl=1  syn_cst_fl=0  syn_cst_dt=unsigned  syn_cst_rnd=on  syn_cst_st=-1  synBlockType=primitive  synLatency=0  synBlockId=15
  Constant1 : shlslibv1/Sources/Constant  syn_cst_val=1  syn_cst_format=Automatic  syn_cst_wl=1  syn_cst_fl=0  syn_cst_dt=unsigned  syn_cst_rnd=on  syn_cst_st=-1  synBlockType=primitive  synLatency=0  synBlockId=15
  Constant2 : shlslibv1/Sources/Constant  syn_cst_val=27  syn_cst_format=Specify  syn_cst_wl=8  syn_cst_fl=0  syn_cst_dt=unsigned  syn_cst_rnd=on  syn_cst_st=-1  synBlockType=primitive  synLatency=0  synBlockId=15
  Extract : shlslibv1/Signal Operations/Extract  syn_extract_vec=[7]  synBlockType=primitive  synLatency=0  synBlockId=17
  Mux : shlslibv1/Signal Operations/Mux  syn_in_nb=2  syn_out_f=Full Precision  syn_out_wl=16  syn_out_fl=8  syn_out_dt=signed  syn_en_se=off  synBlockType=primitive  synLatency=0  synBlockId=16
  Shifter : shlslibv1/Math Functions/Shifter  syn_shifter_opr=<<  syn_out_f=Automatic  syn_out_wl=16  syn_out_fl=8  syn_out_dt=signed  synBlockType=primitive  synLatency=0  synBlockId=12
  Out1 : Outport
  wires:
  Extract/1 -> Comparator/1
  In1/1 -> Shifter/1, Extract/1
  Constant/1 -> Shifter/2
  Constant1/1 -> Comparator/2
  Shifter/1 -> Mux/2, Binary Logic/1
  Comparator/1 -> Mux/1
  Mux/1 -> Out1/1
  Binary Logic/1 -> Mux/3
  Constant2/1 -> Binary Logic/2

== system unrolled_pipelined_parallel/Subsystem/Subsystem4/SB_rs_MIX_COLUMN/Subsystem/multby2 ==
  In1 : Inport
  Binary Logic : shlslibv1/Math Functions/Binary Logic  syn_binlog_exp=a^b  synBlockType=primitive  synLatency=0  synBlockId=13
  Comparator : shlslibv1/Math Functions/Comparator  syn_comp_opr=a==b  syn_comp_const=off  syn_comp_val=0  syn_en_se=off  synBlockType=primitive  synLatency=0  synBlockId=14
  Constant : shlslibv1/Sources/Constant  syn_cst_val=1  syn_cst_format=Automatic  syn_cst_wl=1  syn_cst_fl=0  syn_cst_dt=unsigned  syn_cst_rnd=on  syn_cst_st=-1  synBlockType=primitive  synLatency=0  synBlockId=15
  Constant1 : shlslibv1/Sources/Constant  syn_cst_val=1  syn_cst_format=Automatic  syn_cst_wl=1  syn_cst_fl=0  syn_cst_dt=unsigned  syn_cst_rnd=on  syn_cst_st=-1  synBlockType=primitive  synLatency=0  synBlockId=15
  Constant2 : shlslibv1/Sources/Constant  syn_cst_val=27  syn_cst_format=Specify  syn_cst_wl=8  syn_cst_fl=0  syn_cst_dt=unsigned  syn_cst_rnd=on  syn_cst_st=-1  synBlockType=primitive  synLatency=0  synBlockId=15
  Extract : shlslibv1/Signal Operations/Extract  syn_extract_vec=[7]  synBlockType=primitive  synLatency=0  synBlockId=17
  Mux : shlslibv1/Signal Operations/Mux  syn_in_nb=2  syn_out_f=Full Precision  syn_out_wl=16  syn_out_fl=8  syn_out_dt=signed  syn_en_se=off  synBlockType=primitive  synLatency=0  synBlockId=16
  Shifter : shlslibv1/Math Functions/Shifter  syn_shifter_opr=<<  syn_out_f=Automatic  syn_out_wl=16  syn_out_fl=8  syn_out_dt=signed  synBlockType=primitive  synLatency=0  synBlockId=12
  Out1 : Outport
  wires:
  Extract/1 -> Comparator/1
  In1/1 -> Shifter/1, Extract/1
  Constant/1 -> Shifter/2
  Constant1/1 -> Comparator/2
  Shifter/1 -> Mux/2, Binary Logic/1
  Comparator/1 -> Mux/1
  Mux/1 -> Out1/1
  Binary Logic/1 -> Mux/3
  Constant2/1 -> Binary Logic/2

== system unrolled_pipelined_parallel/Subsystem/Subsystem4/SB_rs_MIX_COLUMN/Subsystem/multby3 ==
  In1 : Inport
  Binary Logic : shlslibv1/Math Functions/Binary Logic  syn_binlog_exp=a^b  synBlockType=primitive  synLatency=0  synBlockId=13
  Comparator : shlslibv1/Math Functions/Comparator  syn_comp_opr=a==b  syn_comp_const=off  syn_comp_val=0  syn_en_se=off  synBlockType=primitive  synLatency=0  synBlockId=14
  Constant : shlslibv1/Sources/Constant  syn_cst_val=1  syn_cst_format=Automatic  syn_cst_wl=1  syn_cst_fl=0  syn_cst_dt=unsigned  syn_cst_rnd=on  syn_cst_st=-1  synBlockType=primitive  synLatency=0  synBlockId=15
  Constant1 : shlslibv1/Sources/Constant  syn_cst_val=1  syn_cst_format=Automatic  syn_cst_wl=1  syn_cst_fl=0  syn_cst_dt=unsigned  syn_cst_rnd=on  syn_cst_st=-1  synBlockType=primitive  synLatency=0  synBlockId=15
  Constant2 : shlslibv1/Sources/Constant  syn_cst_val=27  syn_cst_format=Specify  syn_cst_wl=8  syn_cst_fl=0  syn_cst_dt=unsigned  syn_cst_rnd=on  syn_cst_st=-1  synBlockType=primitive  synLatency=0  synBlockId=15
  Extract : shlslibv1/Signal Operations/Extract  syn_extract_vec=[7]  synBlockType=primitive  synLatency=0  synBlockId=17
  Mux : shlslibv1/Signal Operations/Mux  syn_in_nb=2  syn_out_f=Full Precision  syn_out_wl=16  syn_out_fl=8  syn_out_dt=signed  syn_en_se=off  synBlockType=primitive  synLatency=0  synBlockId=16
  Shifter : shlslibv1/Math Functions/Shifter  syn_shifter_opr=<<  syn_out_f=Automatic  syn_out_wl=16  syn_out_fl=8  syn_out_dt=signed  synBlockType=primitive  synLatency=0  synBlockId=12
  Out1 : Outport
  wires:
  Extract/1 -> Comparator/1
  In1/1 -> Shifter/1, Extract/1
  Constant/1 -> Shifter/2
  Constant1/1 -> Comparator/2
  Shifter/1 -> Mux/2, Binary Logic/1
  Comparator/1 -> Mux/1
  Mux/1 -> Out1/1
  Binary Logic/1 -> Mux/3
  Constant2/1 -> Binary Logic/2

== system unrolled_pipelined_parallel/Subsystem/Subsystem4/SB_rs_MIX_COLUMN/Subsystem/multby4 ==
  In1 : Inport
  Binary Logic : shlslibv1/Math Functions/Binary Logic  syn_binlog_exp=a^b  synBlockType=primitive  synLatency=0  synBlockId=13
  Comparator : shlslibv1/Math Functions/Comparator  syn_comp_opr=a==b  syn_comp_const=off  syn_comp_val=0  syn_en_se=off  synBlockType=primitive  synLatency=0  synBlockId=14
  Constant : shlslibv1/Sources/Constant  syn_cst_val=1  syn_cst_format=Automatic  syn_cst_wl=1  syn_cst_fl=0  syn_cst_dt=unsigned  syn_cst_rnd=on  syn_cst_st=-1  synBlockType=primitive  synLatency=0  synBlockId=15
  Constant1 : shlslibv1/Sources/Constant  syn_cst_val=1  syn_cst_format=Automatic  syn_cst_wl=1  syn_cst_fl=0  syn_cst_dt=unsigned  syn_cst_rnd=on  syn_cst_st=-1  synBlockType=primitive  synLatency=0  synBlockId=15
  Constant2 : shlslibv1/Sources/Constant  syn_cst_val=27  syn_cst_format=Specify  syn_cst_wl=8  syn_cst_fl=0  syn_cst_dt=unsigned  syn_cst_rnd=on  syn_cst_st=-1  synBlockType=primitive  synLatency=0  synBlockId=15
  Extract : shlslibv1/Signal Operations/Extract  syn_extract_vec=[7]  synBlockType=primitive  synLatency=0  synBlockId=17
  Mux : shlslibv1/Signal Operations/Mux  syn_in_nb=2  syn_out_f=Full Precision  syn_out_wl=16  syn_out_fl=8  syn_out_dt=signed  syn_en_se=off  synBlockType=primitive  synLatency=0  synBlockId=16
  Shifter : shlslibv1/Math Functions/Shifter  syn_shifter_opr=<<  syn_out_f=Automatic  syn_out_wl=16  syn_out_fl=8  syn_out_dt=signed  synBlockType=primitive  synLatency=0  synBlockId=12
  Out1 : Outport
  wires:
  Extract/1 -> Comparator/1
  In1/1 -> Shifter/1, Extract/1
  Constant/1 -> Shifter/2
  Constant1/1 -> Comparator/2
  Shifter/1 -> Mux/2, Binary Logic/1
  Comparator/1 -> Mux/1
  Mux/1 -> Out1/1
  Binary Logic/1 -> Mux/3
  Constant2/1 -> Binary Logic/2

== system unrolled_pipelined_parallel/Subsystem/Subsystem4/SB_rs_MIX_COLUMN/Subsystem/multby5 ==
  In1 : Inport
  Binary Logic : shlslibv1/Math Functions/Binary Logic  syn_binlog_exp=a^b  synBlockType=primitive  synLatency=0  synBlockId=13
  Comparator : shlslibv1/Math Functions/Comparator  syn_comp_opr=a==b  syn_comp_const=off  syn_comp_val=0  syn_en_se=off  synBlockType=primitive  synLatency=0  synBlockId=14
  Constant : shlslibv1/Sources/Constant  syn_cst_val=1  syn_cst_format=Automatic  syn_cst_wl=1  syn_cst_fl=0  syn_cst_dt=unsigned  syn_cst_rnd=on  syn_cst_st=-1  synBlockType=primitive  synLatency=0  synBlockId=15
  Constant1 : shlslibv1/Sources/Constant  syn_cst_val=1  syn_cst_format=Automatic  syn_cst_wl=1  syn_cst_fl=0  syn_cst_dt=unsigned  syn_cst_rnd=on  syn_cst_st=-1  synBlockType=primitive  synLatency=0  synBlockId=15
  Constant2 : shlslibv1/Sources/Constant  syn_cst_val=27  syn_cst_format=Specify  syn_cst_wl=8  syn_cst_fl=0  syn_cst_dt=unsigned  syn_cst_rnd=on  syn_cst_st=-1  synBlockType=primitive  synLatency=0  synBlockId=15
  Extract : shlslibv1/Signal Operations/Extract  syn_extract_vec=[7]  synBlockType=primitive  synLatency=0  synBlockId=17
  Mux : shlslibv1/Signal Operations/Mux  syn_in_nb=2  syn_out_f=Full Precision  syn_out_wl=16  syn_out_fl=8  syn_out_dt=signed  syn_en_se=off  synBlockType=primitive  synLatency=0  synBlockId=16
  Shifter : shlslibv1/Math Functions/Shifter  syn_shifter_opr=<<  syn_out_f=Automatic  syn_out_wl=16  syn_out_fl=8  syn_out_dt=signed  synBlockType=primitive  synLatency=0  synBlockId=12
  Out1 : Outport
  wires:
  Extract/1 -> Comparator/1
  In1/1 -> Shifter/1, Extract/1
  Constant/1 -> Shifter/2
  Constant1/1 -> Comparator/2
  Shifter/1 -> Mux/2, Binary Logic/1
  Comparator/1 -> Mux/1
  Mux/1 -> Out1/1
  Binary Logic/1 -> Mux/3
  Constant2/1 -> Binary Logic/2

== system unrolled_pipelined_parallel/Subsystem/Subsystem4/SB_rs_MIX_COLUMN/Subsystem/multby6 ==
  In1 : Inport
  Binary Logic : shlslibv1/Math Functions/Binary Logic  syn_binlog_exp=a^b  synBlockType=primitive  synLatency=0  synBlockId=13
  Comparator : shlslibv1/Math Functions/Comparator  syn_comp_opr=a==b  syn_comp_const=off  syn_comp_val=0  syn_en_se=off  synBlockType=primitive  synLatency=0  synBlockId=14
  Constant : shlslibv1/Sources/Constant  syn_cst_val=1  syn_cst_format=Automatic  syn_cst_wl=1  syn_cst_fl=0  syn_cst_dt=unsigned  syn_cst_rnd=on  syn_cst_st=-1  synBlockType=primitive  synLatency=0  synBlockId=15
  Constant1 : shlslibv1/Sources/Constant  syn_cst_val=1  syn_cst_format=Automatic  syn_cst_wl=1  syn_cst_fl=0  syn_cst_dt=unsigned  syn_cst_rnd=on  syn_cst_st=-1  synBlockType=primitive  synLatency=0  synBlockId=15
  Constant2 : shlslibv1/Sources/Constant  syn_cst_val=27  syn_cst_format=Specify  syn_cst_wl=8  syn_cst_fl=0  syn_cst_dt=unsigned  syn_cst_rnd=on  syn_cst_st=-1  synBlockType=primitive  synLatency=0  synBlockId=15
  Extract : shlslibv1/Signal Operations/Extract  syn_extract_vec=[7]  synBlockType=primitive  synLatency=0  synBlockId=17
  Mux : shlslibv1/Signal Operations/Mux  syn_in_nb=2  syn_out_f=Full Precision  syn_out_wl=16  syn_out_fl=8  syn_out_dt=signed  syn_en_se=off  synBlockType=primitive  synLatency=0  synBlockId=16
  Shifter : shlslibv1/Math Functions/Shifter  syn_shifter_opr=<<  syn_out_f=Automatic  syn_out_wl=16  syn_out_fl=8  syn_out_dt=signed  synBlockType=primitive  synLatency=0  synBlockId=12
  Out1 : Outport
  wires:
  Extract/1 -> Comparator/1
  In1/1 -> Shifter/1, Extract/1
  Constant/1 -> Shifter/2
  Constant1/1 -> Comparator/2
  Shifter/1 -> Mux/2, Binary Logic/1
  Comparator/1 -> Mux/1
  Mux/1 -> Out1/1
  Binary Logic/1 -> Mux/3
  Constant2/1 -> Binary Logic/2

== system unrolled_pipelined_parallel/Subsystem/Subsystem4/SB_rs_MIX_COLUMN/Subsystem/multby7 ==
  In1 : Inport
  Binary Logic : shlslibv1/Math Functions/Binary Logic  syn_binlog_exp=a^b  synBlockType=primitive  synLatency=0  synBlockId=13
  Comparator : shlslibv1/Math Functions/Comparator  syn_comp_opr=a==b  syn_comp_const=off  syn_comp_val=0  syn_en_se=off  synBlockType=primitive  synLatency=0  synBlockId=14
  Constant : shlslibv1/Sources/Constant  syn_cst_val=1  syn_cst_format=Automatic  syn_cst_wl=1  syn_cst_fl=0  syn_cst_dt=unsigned  syn_cst_rnd=on  syn_cst_st=-1  synBlockType=primitive  synLatency=0  synBlockId=15
  Constant1 : shlslibv1/Sources/Constant  syn_cst_val=1  syn_cst_format=Automatic  syn_cst_wl=1  syn_cst_fl=0  syn_cst_dt=unsigned  syn_cst_rnd=on  syn_cst_st=-1  synBlockType=primitive  synLatency=0  synBlockId=15
  Constant2 : shlslibv1/Sources/Constant  syn_cst_val=27  syn_cst_format=Specify  syn_cst_wl=8  syn_cst_fl=0  syn_cst_dt=unsigned  syn_cst_rnd=on  syn_cst_st=-1  synBlockType=primitive  synLatency=0  synBlockId=15
  Extract : shlslibv1/Signal Operations/Extract  syn_extract_vec=[7]  synBlockType=primitive  synLatency=0  synBlockId=17
  Mux : shlslibv1/Signal Operations/Mux  syn_in_nb=2  syn_out_f=Full Precision  syn_out_wl=16  syn_out_fl=8  syn_out_dt=signed  syn_en_se=off  synBlockType=primitive  synLatency=0  synBlockId=16
  Shifter : shlslibv1/Math Functions/Shifter  syn_shifter_opr=<<  syn_out_f=Automatic  syn_out_wl=16  syn_out_fl=8  syn_out_dt=signed  synBlockType=primitive  synLatency=0  synBlockId=12
  Out1 : Outport
  wires:
  Extract/1 -> Comparator/1
  In1/1 -> Shifter/1, Extract/1
  Constant/1 -> Shifter/2
  Constant1/1 -> Comparator/2
  Shifter/1 -> Mux/2, Binary Logic/1
  Comparator/1 -> Mux/1
  Mux/1 -> Out1/1
  Binary Logic/1 -> Mux/3
  Constant2/1 -> Binary Logic/2

== system unrolled_pipelined_parallel/Subsystem/Subsystem4/SB_rs_MIX_COLUMN/Subsystem/multby8 ==
  In1 : Inport
  Binary Logic : shlslibv1/Math Functions/Binary Logic  syn_binlog_exp=a^b  synBlockType=primitive  synLatency=0  synBlockId=13
  Comparator : shlslibv1/Math Functions/Comparator  syn_comp_opr=a==b  syn_comp_const=off  syn_comp_val=0  syn_en_se=off  synBlockType=primitive  synLatency=0  synBlockId=14
  Constant : shlslibv1/Sources/Constant  syn_cst_val=1  syn_cst_format=Automatic  syn_cst_wl=1  syn_cst_fl=0  syn_cst_dt=unsigned  syn_cst_rnd=on  syn_cst_st=-1  synBlockType=primitive  synLatency=0  synBlockId=15
  Constant1 : shlslibv1/Sources/Constant  syn_cst_val=1  syn_cst_format=Automatic  syn_cst_wl=1  syn_cst_fl=0  syn_cst_dt=unsigned  syn_cst_rnd=on  syn_cst_st=-1  synBlockType=primitive  synLatency=0  synBlockId=15
  Constant2 : shlslibv1/Sources/Constant  syn_cst_val=27  syn_cst_format=Specify  syn_cst_wl=8  syn_cst_fl=0  syn_cst_dt=unsigned  syn_cst_rnd=on  syn_cst_st=-1  synBlockType=primitive  synLatency=0  synBlockId=15
  Extract : shlslibv1/Signal Operations/Extract  syn_extract_vec=[7]  synBlockType=primitive  synLatency=0  synBlockId=17
  Mux : shlslibv1/Signal Operations/Mux  syn_in_nb=2  syn_out_f=Full Precision  syn_out_wl=16  syn_out_fl=8  syn_out_dt=signed  syn_en_se=off  synBlockType=primitive  synLatency=0  synBlockId=16
  Shifter : shlslibv1/Math Functions/Shifter  syn_shifter_opr=<<  syn_out_f=Automatic  syn_out_wl=16  syn_out_fl=8  syn_out_dt=signed  synBlockType=primitive  synLatency=0  synBlockId=12
  Out1 : Outport
  wires:
  Extract/1 -> Comparator/1
  In1/1 -> Shifter/1, Extract/1
  Constant/1 -> Shifter/2
  Constant1/1 -> Comparator/2
  Shifter/1 -> Mux/2, Binary Logic/1
  Comparator/1 -> Mux/1
  Mux/1 -> Out1/1
  Binary Logic/1 -> Mux/3
  Constant2/1 -> Binary Logic/2

== system unrolled_pipelined_parallel/Subsystem/Subsystem4/SB_rs_MIX_COLUMN/Subsystem1/multby1 ==
  In1 : Inport
  Binary Logic : shlslibv1/Math Functions/Binary Logic  syn_binlog_exp=a^b  synBlockType=primitive  synLatency=0  synBlockId=13
  Comparator : shlslibv1/Math Functions/Comparator  syn_comp_opr=a==b  syn_comp_const=off  syn_comp_val=0  syn_en_se=off  synBlockType=primitive  synLatency=0  synBlockId=14
  Constant : shlslibv1/Sources/Constant  syn_cst_val=1  syn_cst_format=Automatic  syn_cst_wl=1  syn_cst_fl=0  syn_cst_dt=unsigned  syn_cst_rnd=on  syn_cst_st=-1  synBlockType=primitive  synLatency=0  synBlockId=15
  Constant1 : shlslibv1/Sources/Constant  syn_cst_val=1  syn_cst_format=Automatic  syn_cst_wl=1  syn_cst_fl=0  syn_cst_dt=unsigned  syn_cst_rnd=on  syn_cst_st=-1  synBlockType=primitive  synLatency=0  synBlockId=15
  Constant2 : shlslibv1/Sources/Constant  syn_cst_val=27  syn_cst_format=Specify  syn_cst_wl=8  syn_cst_fl=0  syn_cst_dt=unsigned  syn_cst_rnd=on  syn_cst_st=-1  synBlockType=primitive  synLatency=0  synBlockId=15
  Extract : shlslibv1/Signal Operations/Extract  syn_extract_vec=[7]  synBlockType=primitive  synLatency=0  synBlockId=17
  Mux : shlslibv1/Signal Operations/Mux  syn_in_nb=2  syn_out_f=Full Precision  syn_out_wl=16  syn_out_fl=8  syn_out_dt=signed  syn_en_se=off  synBlockType=primitive  synLatency=0  synBlockId=16
  Shifter : shlslibv1/Math Functions/Shifter  syn_shifter_opr=<<  syn_out_f=Automatic  syn_out_wl=16  syn_out_fl=8  syn_out_dt=signed  synBlockType=primitive  synLatency=0  synBlockId=12
  Out1 : Outport
  wires:
  Extract/1 -> Comparator/1
  In1/1 -> Shifter/1, Extract/1
  Constant/1 -> Shifter/2
  Constant1/1 -> Comparator/2
  Shifter/1 -> Mux/2, Binary Logic/1
  Comparator/1 -> Mux/1
  Mux/1 -> Out1/1
  Binary Logic/1 -> Mux/3
  Constant2/1 -> Binary Logic/2

== system unrolled_pipelined_parallel/Subsystem/Subsystem4/SB_rs_MIX_COLUMN/Subsystem1/multby2 ==
  In1 : Inport
  Binary Logic : shlslibv1/Math Functions/Binary Logic  syn_binlog_exp=a^b  synBlockType=primitive  synLatency=0  synBlockId=13
  Comparator : shlslibv1/Math Functions/Comparator  syn_comp_opr=a==b  syn_comp_const=off  syn_comp_val=0  syn_en_se=off  synBlockType=primitive  synLatency=0  synBlockId=14
  Constant : shlslibv1/Sources/Constant  syn_cst_val=1  syn_cst_format=Automatic  syn_cst_wl=1  syn_cst_fl=0  syn_cst_dt=unsigned  syn_cst_rnd=on  syn_cst_st=-1  synBlockType=primitive  synLatency=0  synBlockId=15
  Constant1 : shlslibv1/Sources/Constant  syn_cst_val=1  syn_cst_format=Automatic  syn_cst_wl=1  syn_cst_fl=0  syn_cst_dt=unsigned  syn_cst_rnd=on  syn_cst_st=-1  synBlockType=primitive  synLatency=0  synBlockId=15
  Constant2 : shlslibv1/Sources/Constant  syn_cst_val=27  syn_cst_format=Specify  syn_cst_wl=8  syn_cst_fl=0  syn_cst_dt=unsigned  syn_cst_rnd=on  syn_cst_st=-1  synBlockType=primitive  synLatency=0  synBlockId=15
  Extract : shlslibv1/Signal Operations/Extract  syn_extract_vec=[7]  synBlockType=primitive  synLatency=0  synBlockId=17
  Mux : shlslibv1/Signal Operations/Mux  syn_in_nb=2  syn_out_f=Full Precision  syn_out_wl=16  syn_out_fl=8  syn_out_dt=signed  syn_en_se=off  synBlockType=primitive  synLatency=0  synBlockId=16
  Shifter : shlslibv1/Math Functions/Shifter  syn_shifter_opr=<<  syn_out_f=Automatic  syn_out_wl=16  syn_out_fl=8  syn_out_dt=signed  synBlockType=primitive  synLatency=0  synBlockId=12
  Out1 : Outport
  wires:
  Extract/1 -> Comparator/1
  In1/1 -> Shifter/1, Extract/1
  Constant/1 -> Shifter/2
  Constant1/1 -> Comparator/2
  Shifter/1 -> Mux/2, Binary Logic/1
  Comparator/1 -> Mux/1
  Mux/1 -> Out1/1
  Binary Logic/1 -> Mux/3
  Constant2/1 -> Binary Logic/2

== system unrolled_pipelined_parallel/Subsystem/Subsystem4/SB_rs_MIX_COLUMN/Subsystem1/multby3 ==
  In1 : Inport
  Binary Logic : shlslibv1/Math Functions/Binary Logic  syn_binlog_exp=a^b  synBlockType=primitive  synLatency=0  synBlockId=13
  Comparator : shlslibv1/Math Functions/Comparator  syn_comp_opr=a==b  syn_comp_const=off  syn_comp_val=0  syn_en_se=off  synBlockType=primitive  synLatency=0  synBlockId=14
  Constant : shlslibv1/Sources/Constant  syn_cst_val=1  syn_cst_format=Automatic  syn_cst_wl=1  syn_cst_fl=0  syn_cst_dt=unsigned  syn_cst_rnd=on  syn_cst_st=-1  synBlockType=primitive  synLatency=0  synBlockId=15
  Constant1 : shlslibv1/Sources/Constant  syn_cst_val=1  syn_cst_format=Automatic  syn_cst_wl=1  syn_cst_fl=0  syn_cst_dt=unsigned  syn_cst_rnd=on  syn_cst_st=-1  synBlockType=primitive  synLatency=0  synBlockId=15
  Constant2 : shlslibv1/Sources/Constant  syn_cst_val=27  syn_cst_format=Specify  syn_cst_wl=8  syn_cst_fl=0  syn_cst_dt=unsigned  syn_cst_rnd=on  syn_cst_st=-1  synBlockType=primitive  synLatency=0  synBlockId=15
  Extract : shlslibv1/Signal Operations/Extract  syn_extract_vec=[7]  synBlockType=primitive  synLatency=0  synBlockId=17
  Mux : shlslibv1/Signal Operations/Mux  syn_in_nb=2  syn_out_f=Full Precision  syn_out_wl=16  syn_out_fl=8  syn_out_dt=signed  syn_en_se=off  synBlockType=primitive  synLatency=0  synBlockId=16
  Shifter : shlslibv1/Math Functions/Shifter  syn_shifter_opr=<<  syn_out_f=Automatic  syn_out_wl=16  syn_out_fl=8  syn_out_dt=signed  synBlockType=primitive  synLatency=0  synBlockId=12
  Out1 : Outport
  wires:
  Extract/1 -> Comparator/1
  In1/1 -> Shifter/1, Extract/1
  Constant/1 -> Shifter/2
  Constant1/1 -> Comparator/2
  Shifter/1 -> Mux/2, Binary Logic/1
  Comparator/1 -> Mux/1
  Mux/1 -> Out1/1
  Binary Logic/1 -> Mux/3
  Constant2/1 -> Binary Logic/2

== system unrolled_pipelined_parallel/Subsystem/Subsystem4/SB_rs_MIX_COLUMN/Subsystem1/multby4 ==
  In1 : Inport
  Binary Logic : shlslibv1/Math Functions/Binary Logic  syn_binlog_exp=a^b  synBlockType=primitive  synLatency=0  synBlockId=13
  Comparator : shlslibv1/Math Functions/Comparator  syn_comp_opr=a==b  syn_comp_const=off  syn_comp_val=0  syn_en_se=off  synBlockType=primitive  synLatency=0  synBlockId=14
  Constant : shlslibv1/Sources/Constant  syn_cst_val=1  syn_cst_format=Automatic  syn_cst_wl=1  syn_cst_fl=0  syn_cst_dt=unsigned  syn_cst_rnd=on  syn_cst_st=-1  synBlockType=primitive  synLatency=0  synBlockId=15
  Constant1 : shlslibv1/Sources/Constant  syn_cst_val=1  syn_cst_format=Automatic  syn_cst_wl=1  syn_cst_fl=0  syn_cst_dt=unsigned  syn_cst_rnd=on  syn_cst_st=-1  synBlockType=primitive  synLatency=0  synBlockId=15
  Constant2 : shlslibv1/Sources/Constant  syn_cst_val=27  syn_cst_format=Specify  syn_cst_wl=8  syn_cst_fl=0  syn_cst_dt=unsigned  syn_cst_rnd=on  syn_cst_st=-1  synBlockType=primitive  synLatency=0  synBlockId=15
  Extract : shlslibv1/Signal Operations/Extract  syn_extract_vec=[7]  synBlockType=primitive  synLatency=0  synBlockId=17
  Mux : shlslibv1/Signal Operations/Mux  syn_in_nb=2  syn_out_f=Full Precision  syn_out_wl=16  syn_out_fl=8  syn_out_dt=signed  syn_en_se=off  synBlockType=primitive  synLatency=0  synBlockId=16
  Shifter : shlslibv1/Math Functions/Shifter  syn_shifter_opr=<<  syn_out_f=Automatic  syn_out_wl=16  syn_out_fl=8  syn_out_dt=signed  synBlockType=primitive  synLatency=0  synBlockId=12
  Out1 : Outport
  wires:
  Extract/1 -> Comparator/1
  In1/1 -> Shifter/1, Extract/1
  Constant/1 -> Shifter/2
  Constant1/1 -> Comparator/2
  Shifter/1 -> Mux/2, Binary Logic/1
  Comparator/1 -> Mux/1
  Mux/1 -> Out1/1
  Binary Logic/1 -> Mux/3
  Constant2/1 -> Binary Logic/2
